simulink model "Sensor_GPS"  (R2016b)
settings: Solver=FixedStepAuto  StartTime=0.0  StopTime=10.0  RelTol=1e-3
libraries: Sensors_Lib x4
settings Model: ParameterArgumentNames=sens  Creator=rega0051  LastModifiedBy=rega0051

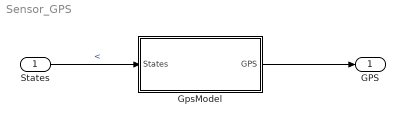
== system Sensor_GPS ==
  "States " : Inport  OutDataTypeStr=Bus: States
  GpsModel : Subsystem  Variant=on  VariantControl=Variant1
  " GPS" : Outport  OutDataTypeStr=Bus: GPS
  wires:
  "States "/1 -> GpsModel/1("States ")  "<"
  GpsModel/1(" GPS") -> " GPS"/1

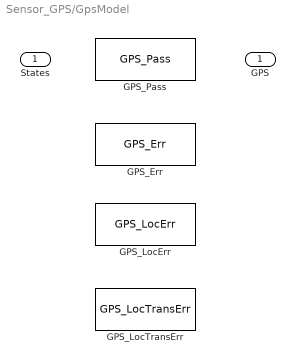
== system Sensor_GPS/GpsModel ==
  "States " : Inport  OutDataTypeStr=Bus: States
  GPS_Err : Sensors_Lib/GPS Sensor Models/GPS_Err  VariantControl=VarGps_Err
  GPS_LocErr : Sensors_Lib/GPS Sensor Models/GPS_LocErr  VariantControl=VarGps_LocErr
  GPS_LocTransErr : Sensors_Lib/GPS Sensor Models/GPS_LocTransErr  VariantControl=VarGps_LocTransErr
  GPS_Pass : Sensors_Lib/GPS Sensor Models/GPS_Pass  VariantControl=VarGps_Pass
  " GPS" : Outport  OutDataTypeStr=Bus: GPS
